simulink library "target_mpc555"  (Simulink 6.0)
settings: Solver=ode45  SolverMode=SingleTasking  StartTime=0.0  StopTime=10.0  RelTol=1e-3
PreLoadFcn:
  | RTWConfigurationCB('preloadfcn', bdroot);
InitFcn:
  | % START RTW CONFIGURATION CODE %
  | RTWConfigurationCB('rtw_target_initfcn',gcs);
  | % END RTW CONFIGURATION CODE %
libraries: driver_interface_library x2, simulink x1, target_mpc555 x1
settings Model: Creator=The MathWorks Inc.  LastModifiedBy=batserve  ExtModeAutoUpdateStatusClock=off  ProdHWDeviceType=Specified
settings DataIOCC: SignalLoggingName=logsOut
settings OptimizationCC: BooleanDataType=off
settings DebuggingCC: CheckExecutionContextPreStartOutputMsg=on  CheckExecutionContextRuntimeOutputMsg=on  SolverPrmCheckMsg=none
settings HardwareCC: ProdHWDeviceType=Specified

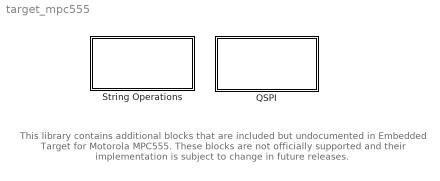
== system target_mpc555 ==
  note: This library contains additional blocks that are included but undocumented in
      | Embedded Target for Motorola MPC555. These blocks are not officially supported
      | and their implementation is subject to change in future releases.
  QSPI : Subsystem  PropExecContextAcrossSSBoundary=on
      mask Type: QSPI
      mask Display: disp('QSPI')
  String Operations : Subsystem  PropExecContextAcrossSSBoundary=on
      mask Display: disp('String Operations');

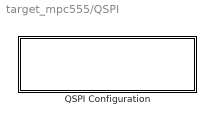
== system target_mpc555/QSPI ==
  QSPI Configuration : Subsystem  Tag=_MPC555_QSPI_CONFIG_  PropExecContextAcrossSSBoundary=on  mask(Queued Serial Peripheral Interface Configuration){irqLevel=INT_LEVEL6, qlen=15}
      mask prompts: irqLevel "IRQ Level"; qlen "Queue Length"
      mask help:
      | MPC555 QSPI configuration block
      |
      | If the QSPI driver is to be used, then there must be exactly one copy of this block within the overall model.
      |
      | The IRQ Level parameter is the MPC555 interrupt level that is used to trigger an interrupt when a transfer is complete. This interrupt is used to check whether any additional QSPI jobs are queued, and if so to startthe highest priority job running.
      |
      | The Queue Length is the length of the queue used to store QSPI jobs that have been submitted and are ready to start.
      mask init:
      | irqLevel = mask_resource_validator(gcb,@mask_qspi_validator, irqLevel);
      mask StyleString: popup(INT_LEVEL0|INT_LEVEL1|INT_LEVEL2|INT_LEVEL3|INT_LEVEL4|INT_LEVEL5|INT_LEVEL6|INT_LEVEL7|INT_LEVEL8|INT_LEVEL9|INT_LEVEL10|INT_LEVEL11|INT_LEVEL12|INT_LEVEL13|INT_LEVEL14|INT_LEVEL15|INT_LEVEL16|INT_LEVEL17|INT_LEVEL18|INT_LEVEL19|INT_LEVEL20|INT_LEVEL21|INT_LEVEL22|INT_LEVEL23|INT_LEVEL24|INT_LEVEL25|INT_LEVEL26|INT_LEVEL27|INT_LEVEL28|INT_LEVEL29|INT_LEVEL30|INT_LEVEL31),edit
      mask Display: disp('MPC555 QSPI Configuration')

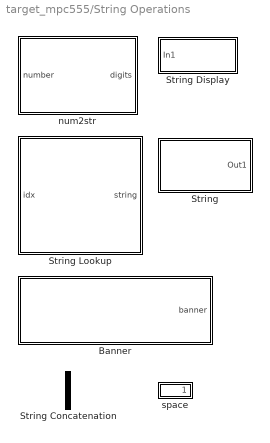
== system target_mpc555/String Operations ==
  Banner : Subsystem  PropExecContextAcrossSSBoundary=on  mask(Banner){banner=Hello This Is My First Banner, t=1, banner_width=10}
      mask prompts: banner "String"; t "Sample Time"; banner_width "Visible Banner Width"
      mask help:
      | The output of this block is a sliding window over the banner string.
      |
      | The output is standard ASCII codes output as a wide uint8 signal.
      mask Display:
      | text(0.5,0.8,[ num2str(banner_width) 'char wide banner' ],'horizontalalignment','center')
      | disp(banner)
      | plot([0.25 0.75 0.75 0.25 0.25],[0.3 0.3 0.7 0.7 0.3])
      | plot([0.25 0.5],[0.1 0.1]);
      | plot([0.4 0.5 0.4 0.4],[0.175 0.1 0.025 0.175])
  String : Subsystem  PropExecContextAcrossSSBoundary=on  mask(String Output){S=A String}
      mask prompts: S "String"
      mask help: Represent the string in standard ASCII code as a wide uint8 signal.
      mask init:
      | u = uint8(S);
      mask Display: disp(S)
  String Concatenation : Mux  Inputs=2
  String Display : Subsystem  PropExecContextAcrossSSBoundary=on  mask(String Display){S=}
      mask help: Displays a vector of characters as a string on the block. The input should be a wide vector. Each element in the vector should be the numerical ASCII code for that character.
      mask init:
      | block=gcb;
      mask Display: disp(S)
  String Lookup : Subsystem  PropExecContextAcrossSSBoundary=on  mask(String Lookup){S={'string1' 'string2' 'string3'  'string4'}}
      mask prompts: S "Strings"
      mask help:
      | Specify a cell array of strings as a lookup table.
      |
      | The input to the block is base zero addressing so the first string will be output if the input is 0. The output is standard ASCII code and will be a wide uint8 vector as wide as the largest string in the cell array set.
      mask init:
      | SS = S;
      | SS = [ sprintf('%s\\n',S{1:end-1}) S{end} ];
      | S = uint8(strvcat(S{:}))';
      | 
      | if size(S,2)<=1
      |    error('You must have at least two strings for the lookup table');
      | end
      mask Display:
      | text(0.1,0.9,'STRING LOOKUP :');
      | text(0.2,0.4,SS)
      | 
      | plot([0.15 0.15],[0 0.8]);
      | plot([0.15 0.5],[0 0])
      | plot([0.15 0.5],[0.8 0.8])
  num2str : Subsystem  TreatAsAtomicUnit=on  PropExecContextAcrossSSBoundary=on  mask(Num2Str){N=6, S=1, O=0, B=10}
      mask prompts: N "Number of digits"; S "Scaling"; O "Offset"; B "Base"
      mask help:
      | Converts an input number to a string output.
      |
      | Given the scaling and offset and the number of digits to output a string is represented in standard ASCII codes as a wide uint8 signal line.
      mask init:
      | if B <=0 | B >10
      |    error('Base must be between 1 and 10');
      | end
      mask Help: Converts an input number to a string output given the scaling and offset and the number of digits to output. The string is output in standard ASCII codes as a wide uint8 signal line.
      mask Display: text(0.1,0.5,sprintf('Number to String\\n   digits      %d\\n   scaling   %g\\n   offset      %g',N,S,O))
  space : Subsystem  PropExecContextAcrossSSBoundary=on
      mask Type: Single White Space
      mask Description: When you mux strings together you can insert this block to make sure there is whitespace between the strings.
      mask Display: disp('''  ''');

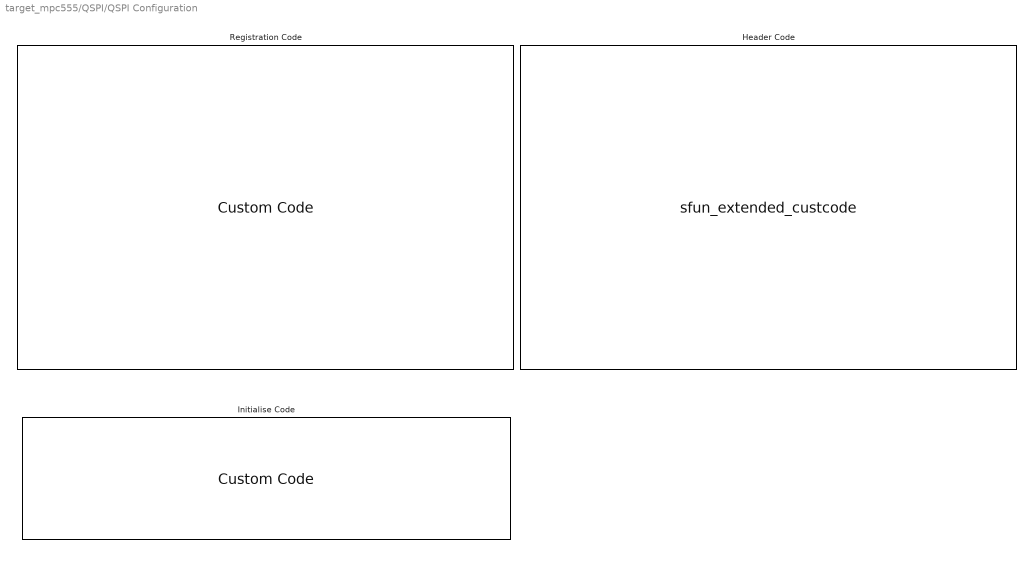
== system target_mpc555/QSPI/QSPI Configuration ==
  Header Code : S-Function  FunctionName=sfun_extended_custcode  mask(Subsystem Custom Coder){}
      mask help: Add code to subsystem Derivatives function
      mask init:
      | [ dispstr,rtwdata ] = mask_custom_code_java('process_code',gcb);
      | set_param(gcb,'rtwdata',rtwdata);
      settings: OpenFcn=mask_custom_code_java('initfcn',gcb)
      mask Help:
      | This block contains text fields to insert custom user code sections at the declaration, execution and exit sections of the subsystem derivatives function.  By placing this block inside a subsytem, the custom user code will appear in that subsystems function. <p>
      | 
      | You can choose to have the code appear only once for all instances of the enclosing masked library block. To activate this option select <b>"Generate once per functional mask"</b> option. This option can be further refined by defining a <b>key</b> For example if there are 4 instances of a library block and two have the key "XX" and two have the key "YY" then the code generation block will generate code once for the "XX" blocks and once for the "YY" blocks.
      mask Display: text(0.1,0.5,dispstr,'horizontalAlignment','left')
  Initialise Code : driver_interface_library/Custom Code
  Registration Code : driver_interface_library/Custom Code

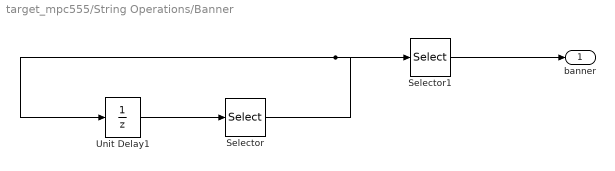
== system target_mpc555/String Operations/Banner ==
  Selector : Selector  Elements=[2:length(banner) 1 ]  InputPortWidth=length(banner)
  Selector1 : Selector  Elements=[1:banner_width]
  Unit Delay1 : UnitDelay  X0=uint8(banner)  SampleTime=t
  banner : Outport
  wires:
  Selector/1 -> Unit Delay1/1, Selector1/1
  Unit Delay1/1 -> Selector/1
  Selector1/1 -> banner/1

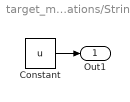
== system target_mpc555/String Operations/String ==
  Constant : Constant  Value=u
  Out1 : Outport
  wires:
  Constant/1 -> Out1/1

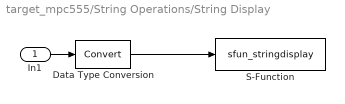
== system target_mpc555/String Operations/String Display ==
  In1 : Inport  Port=1  LatchInput=off
  Data Type Conversion : DataTypeConversion  SaturateOnIntegerOverflow=on  RndMeth=Zero
  S-Function : S-Function  FunctionName=sfun_stringdisplay  Parameters=block  mask{block=block, S=1}
      mask Display: disp(S)
  wires:
  In1/1 -> Data Type Conversion/1
  Data Type Conversion/1 -> S-Function/1

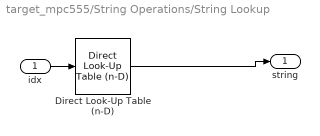
== system target_mpc555/String Operations/String Lookup ==
  idx : Inport  Port=1  LatchInput=off
  Direct Look-Up Table (n-D) : simulink/Look-Up Tables/Direct Look-Up Table (n-D)  maskTabDims=2  explicitNumDims=1  outDims=Column  tabIsInput=off  mxTable=S  clipFlag=Warning
  string : Outport
  wires:
  idx/1 -> Direct Look-Up Table (n-D)/1
  Direct Look-Up Table (n-D)/1 -> string/1

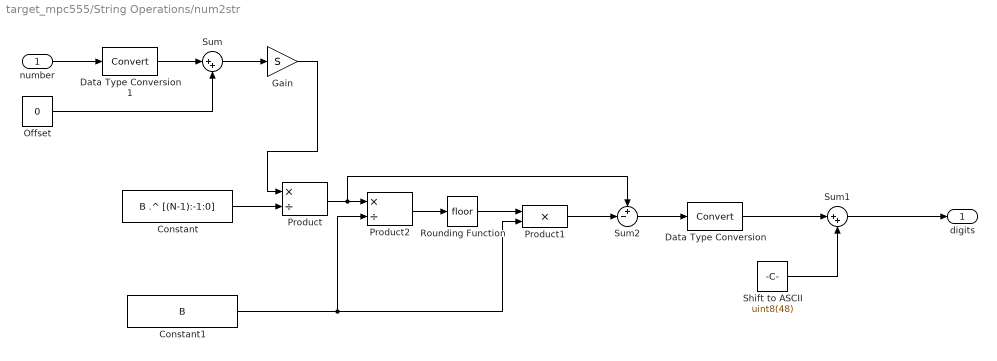
== system target_mpc555/String Operations/num2str ==
  number : Inport  Port=1  LatchInput=off
  Constant : Constant  Value=B .^ [(N-1):-1:0]
  Constant1 : Constant  Value=B
  Data Type Conversion : DataTypeConversion  RndMeth=Zero
  Data Type Conversion1 : DataTypeConversion  RndMeth=Zero
  Gain : Gain  Gain=S  SaturateOnIntegerOverflow=on
  Offset : Constant  Value=0
  Product : Product  Inputs=*/  SaturateOnIntegerOverflow=on  InputSameDT=on
  Product1 : Product  Inputs=**  SaturateOnIntegerOverflow=on  InputSameDT=on
  Product2 : Product  Inputs=*/  SaturateOnIntegerOverflow=on  InputSameDT=on
  Rounding Function : Rounding
  Shift to ASCII : Constant  Value=uint8(48)
  Sum : Sum  Inputs=|++  SaturateOnIntegerOverflow=on  InputSameDT=on
  Sum1 : Sum  Inputs=|++  InputSameDT=on
  Sum2 : Sum  Inputs=+-|  InputSameDT=on
  digits : Outport
  wires:
  Product1/1 -> Sum2/2
  Constant1/1 -> Product1/2, Product2/2
  Constant/1 -> Product/2
  number/1 -> Data Type Conversion1/1
  Sum/1 -> Gain/1
  Offset/1 -> Sum/2
  Gain/1 -> Product/1
  Sum1/1 -> digits/1
  Shift to ASCII/1 -> Sum1/2
  Data Type Conversion1/1 -> Sum/1
  Rounding Function/1 -> Product1/1
  Product/1 -> Product2/1, Sum2/1
  Product2/1 -> Rounding Function/1
  Sum2/1 -> Data Type Conversion/1
  Data Type Conversion/1 -> Sum1/1

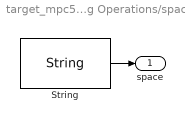
== system target_mpc555/String Operations/space ==
  String : target_mpc555/String Operations/String  S=""
  space : Outport
  wires:
  String/1 -> space/1
